simulink model "mychapter5"  (R2022b)
settings: Solver=ode45  StartTime=0.0  StopTime=40  FixedStep=0.01  RelTol=1e-3  EnableMultiTasking=on
libraries: Solver_SF x1
settings Model: Creator=xuwei  LastModifiedBy=wyx
settings SolverCC: AlgebraicLoopSolver=TrustRegion
settings DataIOCC: LimitDataPoints=on  SaveFormat=Array  SignalLoggingSaveFormat=ModelDataLogs  ReturnWorkspaceOutputs=off
settings OptimizationCC: ExpressionDepthLimit=2147483647  LifeSpan=inf
settings DebuggingCC: UnderspecifiedInitializationDetection=Classic  MergeDetectMultiDrivingBlocksExec=none  SolverPrmCheckMsg=warning  FcnCallInpInsideContextMsg=warning  UnconnectedInputMsg=warning  UnconnectedOutputMsg=warning  UnconnectedLineMsg=warning  StateNameClashWarn=warning  SFUnexpectedBacktrackingDiag=warning  SFNoUnconditionalDefaultTransitionDiag=warning  SFExecutionAtInitializationDiag=none  SFMachineParentedDataDiag=warning  ArithmeticOperatorsInVariantConditions=warning
settings HardwareCC: ProdBitPerPointer=32  ProdBitPerSizeT=32  ProdBitPerPtrDiffT=32  ProdLargestAtomicFloat=None  ProdIntDivRoundTo=Undefined  ProdEndianess=Unspecified  ProdWordSize=32  ProdHWDeviceType=32-bit Generic
settings ModelReferenceCC: PropagateSignalLabelsOutOfModel=off
settings SFSimCC: SimUseLocalCustomCode=off  CustomCodeUndefinedFunction=UseInterfaceOnly
settings RTWCC: RTWUseLocalCustomCode=off
settings CodeAppCC: StateflowObjectComments=on
settings GRTTargetCC: TargetLangStandard=C89/C90 (ANSI)  CombineOutputUpdateFcns=off  GRTInterface=on
settings ConfigComp: CovMetricSettings=dw  CovSaveCumulativeToWorkspaceVar=on  CovSaveSingleToWorkspaceVar=on  CovExternalEMLEnable=off
settings SimscapeCC: SimscapeNormalizeSystem=off
settings ConfigurationSet: Description=SimMechanics 2G

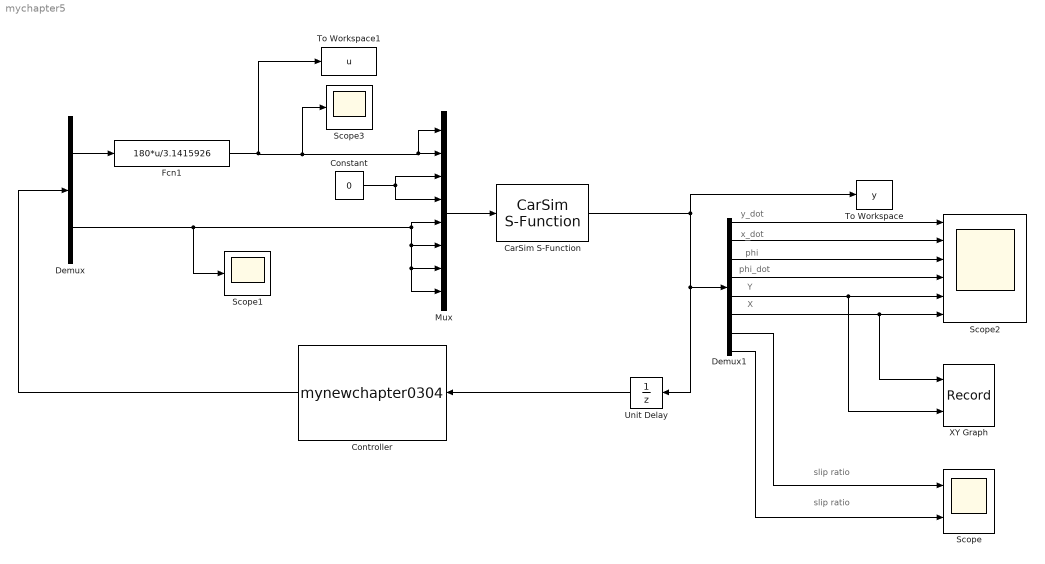
== system mychapter5 ==
  note: y_dot
  note: x_dot
  note: phi
  note: phi_dot
  note: Y
  note: X
  note: slip ratio
  note: slip ratio
  CarSim S-Function : Solver_SF/CarSim S-Function  Priority=1  SIMFILE=simfile.sim
  Constant : Constant  Value=0
  Controller : S-Function  FunctionName=mynewchapter0304  SFunctionDeploymentMode=off  EnableBusSupport=off
  Demux : Demux  Outputs=2
  Demux1 : Demux  Outputs=8
  Fcn1 : Fcn  Expr=180*u/3.1415926
  Mux : Mux  Inputs=8
  Scope : Scope  NumInputPorts=2
  Scope1 : Scope
  Scope2 : Scope  NumInputPorts=6
  Scope3 : Scope
  To Workspace : ToWorkspace  VariableName=y  SaveFormat=Structure  SampleTime=-1
  To Workspace1 : ToWorkspace  VariableName=u  SaveFormat=Structure  SampleTime=-1
  Unit Delay : UnitDelay  SampleTime=-1  HasFrameUpgradeWarning=on
  XY Graph : Record  FileSettingsInternal="{\"entries\":[{\"content\":{\"excelSettings\":{\"content\":{},\"type\":\"Streamout.ExcelSettings\"}},\"type\":\"Streamout.FileSettingStorage\",\"uuid\":\"3260fb28-714c-40a1-9467-384836d80718\"}],\"packageUris\":[\"http://schema.mathworks.com/mf0/streamout_blocks/R2020a\"],\"version\":\"1.0\"}"  Layout=[1 1]  SignalsInternal="{\"entries\":[{\"content\":{\"signals\":[{\"content\":{\"blockPath\":[\"mychapter5/XY Graph\"],\"channel\":[],\"dimensions\":[1],\"domain\":\"mychapter5/XY Graph\",\"lineColor\":\"#a2142f\",\"plots\":[],\"port\":1,\"sid\":[\"\"],\"signalID\":636,\"signalName\":\"Demux1:6\"},\"type\":\"RecordBlkView.Signal\",\"uuid\":\"bb4ffeb7-3682-45a0-8da7-a2546fcb3904\"},{\"content\":{\"blockPath\":[\"mychapter5/XY Graph\"],\"channel\":[],\"dimensions\":[1],\"domain\":\"mychapter5/XY Graph\",\"lineColor\":\"#139fff\",\"plots\":[],\"port\":2,\"sid\":[\"\"],\"signalID\":640,\"signalName\":\"Demux1:5\"},\"type\":\"RecordBlkView.Signal\",\"uuid\":\"ae240acd-8cde-4928-9545-1565a2596212\"}]},\"type\":\"RecordBlkView.InputSignals\",\"uuid\":\"51186d5f-65eb-4d81-96d6-199ef0d56072\"}],\"packageUris\":[\"http://schema.mathworks.com/mf0/streamout_blocks/R2020a\"],\"version\":\"1.0\"}"  VisualizationBindings="{\"xyplotplugin\":{\"info\":[{\"series\":[],\"subplotID\":1}]}}"  CompatibilityTag=XY  st=-1
  wires:
  CarSim S-Function/1 -> To Workspace/1, Unit Delay/1, Demux1/1
  Demux1/1 -> Scope2/1
  Demux1/2 -> Scope2/2
  Demux1/3 -> Scope2/3
  Demux1/4 -> Scope2/4
  Demux1/5 -> XY Graph/2, Scope2/5
  Demux1/6 -> XY Graph/1, Scope2/6
  Unit Delay/1 -> Controller/1
  Demux1/7 -> Scope/1
  Demux1/8 -> Scope/2
  Mux/1 -> CarSim S-Function/1
  Constant/1 -> Mux/4, Mux/3
  Fcn1/1 -> Scope3/1, Mux/1, Mux/2, To Workspace1/1
  Demux/2 -> Scope1/1, Mux/5, Mux/8, Mux/7, Mux/6
  Controller/1 -> Demux/1
  Demux/1 -> Fcn1/1
